simulink subsystem "moiVariant"  (R2023a)
settings: Solver=VariableStepAuto  StartTime=0.0  StopTime=10.0  RelTol=1e-3
settings Model: Creator=KozlovM  LastModifiedBy=diontep

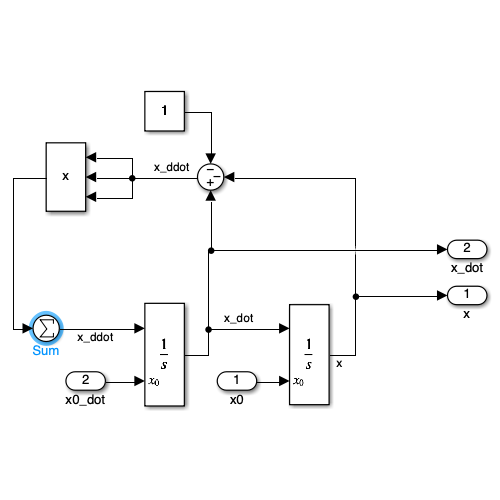
[thumbnail: Simulink's stored preview of the top-level diagram]
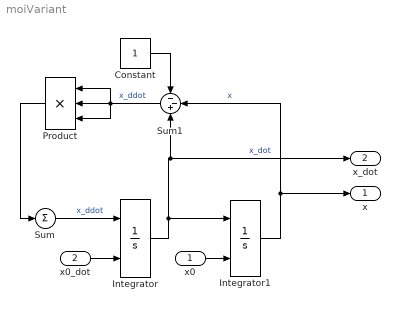
== system moiVariant ==
  x0 : Inport
  x0_dot : Inport  Port=2
  Constant : Constant
  Integrator : Integrator  InitialConditionSource=external
  Integrator1 : Integrator  InitialConditionSource=external
  Product : Product  Inputs=3
  Sum : Sum  Inputs=+
  Sum1 : Sum  Inputs=--+
  x : Outport
  x_dot : Outport  Port=2
  wires:
  Integrator1/1 -> Sum1/2, x/1  "x"
  Integrator/1 -> Integrator1/1, x_dot/1, Sum1/3  "x_dot"
  x0_dot/1 -> Integrator/2
  x0/1 -> Integrator1/2
  Sum/1 -> Integrator/1  "x_ddot"
  Product/1 -> Sum/1
  Sum1/1 -> Product/3, Product/2, Product/1  "x_ddot"
  Constant/1 -> Sum1/1
